simulink model "model_statex"  (R2016a)
settings: Solver=VariableStepAuto  StartTime=0.0  StopTime=10.0  RelTol=1e-3
values from neighbouring files (symbols this model uses):
  A = [-5 -3 0;-4 -2.5 0;0 1 0]    [Model_C1.m]
  B = [0.15;-0.1;0]    [Model_C1.m]
  C = [0 0 1]    [Model_C1.m]
  K = acker(A, B, Pcom)    [Model_C1.m]
  L = acker(A', C', Pobs)    [Model_C1.m]
  Nbar = 1    [Model_C1.m]
  Step_final = 1    [Model_C1.m]
settings Model: Creator=massona  LastModifiedBy=massona

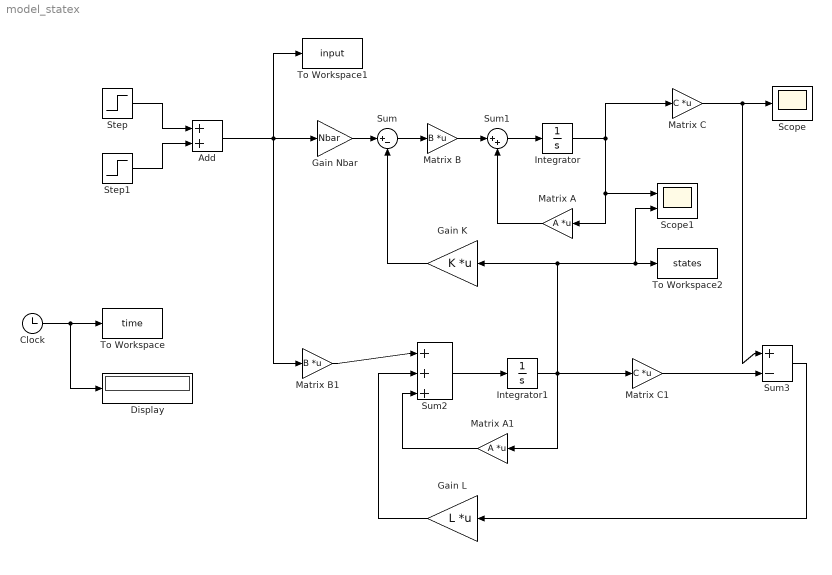
== system model_statex ==
  Add : Sum
  Clock : Clock
  Display : Display
  Gain K : Gain  Gain=K  Multiplication=Matrix(K*u) (u vector)
  Gain L : Gain  Gain=L  Multiplication=Matrix(K*u) (u vector)
  Gain Nbar : Gain  Gain=Nbar
  Integrator : Integrator
  Integrator1 : Integrator
  Matrix A : Gain  Gain=A  Multiplication=Matrix(K*u)
  Matrix A1 : Gain  Gain=A  Multiplication=Matrix(K*u)
  Matrix B : Gain  Gain=B  Multiplication=Matrix(K*u)
  Matrix B1 : Gain  Gain=B  Multiplication=Matrix(K*u)
  Matrix C : Gain  Gain=C  Multiplication=Matrix(K*u)
  Matrix C1 : Gain  Gain=C  Multiplication=Matrix(K*u)
  Scope : Scope
  Scope1 : Scope  NumInputPorts=2
  Step : Step  After=Step_final  SampleTime=0
  Step1 : Step  Time=6  After=-Step_final  SampleTime=0
  Sum : Sum  Inputs=|+-
  Sum1 : Sum  Inputs=|++
  Sum2 : Sum  Inputs=|+++
  Sum3 : Sum  Inputs=|+-
  To Workspace : ToWorkspace  VariableName=time  SampleTime=-1
  To Workspace1 : ToWorkspace  VariableName=input  SampleTime=-1
  To Workspace2 : ToWorkspace  VariableName=states  SampleTime=-1
  wires:
  Step/1 -> Add/1
  Step1/1 -> Add/2
  Clock/1 -> Display/1, To Workspace/1
  Add/1 -> Matrix B1/1, Gain Nbar/1, To Workspace1/1
  Gain Nbar/1 -> Sum/1
  Sum/1 -> Matrix B/1
  Matrix B/1 -> Sum1/1
  Sum1/1 -> Integrator/1
  Integrator/1 -> Matrix C/1, Matrix A/1, Scope1/1
  Matrix A/1 -> Sum1/2
  Gain K/1 -> Sum/2
  Matrix C/1 -> Sum3/1, Scope/1
  Matrix B1/1 -> Sum2/1
  Sum2/1 -> Integrator1/1
  Integrator1/1 -> Scope1/2, To Workspace2/1, Gain K/1, Matrix C1/1, Matrix A1/1
  Matrix A1/1 -> Sum2/3
  Matrix C1/1 -> Sum3/2
  Gain L/1 -> Sum2/2
  Sum3/1 -> Gain L/1
